simulink model "bolita_sim_2018a"  (R2018a)
settings: Solver=VariableStepAuto  StartTime=0.0  StopTime=10  RelTol=1e-3
values from neighbouring files (symbols this model uses):
  A = double(subs(A,{x1,x2,x3,u},{x1_eq,x2_eq,x3_eq,u_eq}))    [bolita.m]
  B = double(subs(B,{x1,x2,x3,u},{x1_eq,x2_eq,x3_eq,u_eq}))    [bolita.m]
  C = double(subs(C,{x1,x2,x3,u},{x1_eq,x2_eq,x3_eq,u_eq}))    [bolita.m]
  Ki = Ki(end)    [bolita.m]
  Ksr = Ki(1:3)    [bolita.m]
  L = (acker(A',C',[-200 -200 -200]))'    [bolita.m]
  u_eq = double(solve(subs(x3_dot,x3,x3_eq)))    [bolita.m]
  x1_eq = 0    [bolita.m]
  x2_eq = 0    [bolita.m]
  x3_eq = double(solve(subs(x2_dot,x1,x1_eq)))    [bolita.m]
settings Model: Creator=Carlos  LastModifiedBy=Carlos
settings DebuggingCC: LibraryContextMissingDiagnostic=warning
settings SFSimCC: SimUseLocalCustomCode=on
settings RTWCC: RTWUseLocalCustomCode=on

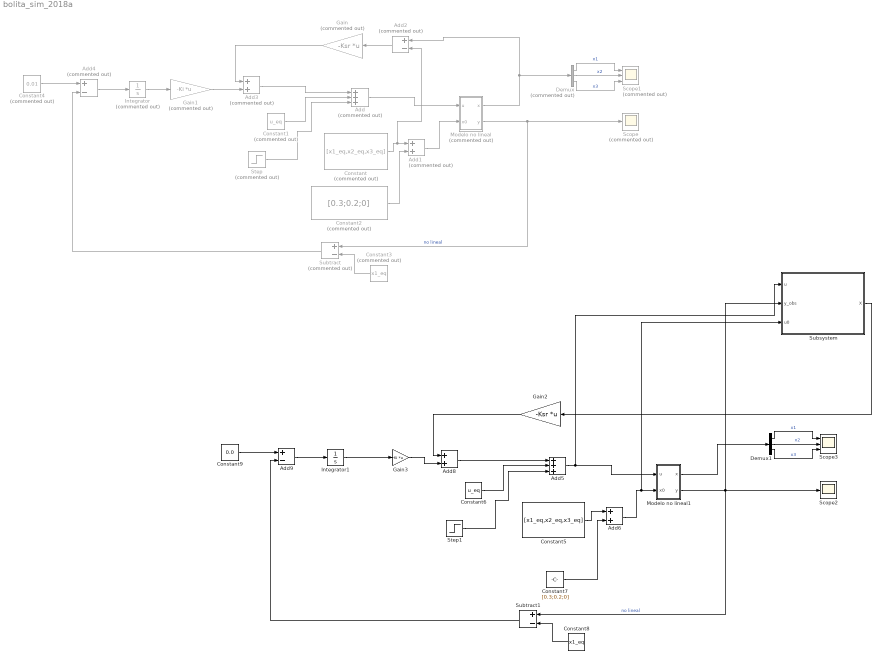
== system bolita_sim_2018a ==
  Add : Sum  Commented=on  Inputs=+++
  Add1 : Sum  Commented=on
  Add2 : Sum  Commented=on  Inputs=+-
  Add3 : Sum  Commented=on
  Add4 : Sum  Commented=on  Inputs=+-
  Add5 : Sum  Inputs=+++
  Add6 : Sum
  Add8 : Sum
  Add9 : Sum  Inputs=+-
  Constant : Constant  Commented=on  Value=[x1_eq,x2_eq,x3_eq]
  Constant1 : Constant  Commented=on  Value=u_eq
  Constant2 : Constant  Commented=on  Value=[0.3;0.2;0]
  Constant3 : Constant  Commented=on  Value=x1_eq
  Constant4 : Constant  Commented=on  Value=0.01
  Constant5 : Constant  Value=[x1_eq,x2_eq,x3_eq]
  Constant6 : Constant  Value=u_eq
  Constant7 : Constant  Value=[0.3;0.2;0]
  Constant8 : Constant  Value=x1_eq
  Constant9 : Constant  Value=0.0
  Demux : Demux  Commented=on  Outputs=3
  Demux1 : Demux  Outputs=3
  Gain : Gain  Commented=on  Gain=-Ksr  Multiplication=Matrix(K*u) (u vector)
  Gain1 : Gain  Commented=on  Gain=-Ki  Multiplication=Matrix(K*u) (u vector)
  Gain2 : Gain  Gain=-Ksr  Multiplication=Matrix(K*u) (u vector)
  Gain3 : Gain  Gain=-Ki  Multiplication=Matrix(K*u) (u vector)
  Integrator : Integrator  Commented=on
  Integrator1 : Integrator
  Modelo no lineal : Subsystem  Commented=on
  Modelo no lineal1 : Subsystem
  Scope : Scope  Commented=on
  Scope1 : Scope  Commented=on  NumInputPorts=3
  Scope2 : Scope
  Scope3 : Scope  NumInputPorts=3
  Step : Step  Commented=on  Time=5  After=300  SampleTime=0
  Step1 : Step  Time=5  After=300  SampleTime=0
  Subsystem : Subsystem
  Subtract : Sum  Commented=on  Inputs=+-
  Subtract1 : Sum  Inputs=+-
  wires:
  Add/1 -> Modelo no lineal/1(u)
  Constant1/1 -> Add/2
  Modelo no lineal/1(x) -> Demux/1, Add2/1
  Constant/1 -> Add2/2, Add1/1
  Add1/1 -> Modelo no lineal/2(x0)
  Constant2/1 -> Add1/2
  Add2/1 -> Gain/1
  Modelo no lineal/2(y) -> Subtract/1, Scope/1  "no lineal"
  Demux/1 -> Scope1/1  "x1"
  Demux/2 -> Scope1/2  "x2"
  Demux/3 -> Scope1/3  "x3"
  Add3/1 -> Add/1
  Gain1/1 -> Add3/2
  Gain/1 -> Add3/1
  Integrator/1 -> Gain1/1
  Constant3/1 -> Subtract/2
  Add4/1 -> Integrator/1
  Subtract/1 -> Add4/2
  Constant4/1 -> Add4/1
  Step/1 -> Add/3
  Subsystem/1(X) -> Gain2/1
  Add8/1 -> Add5/1
  Step1/1 -> Add5/3
  Add9/1 -> Integrator1/1
  Demux1/3 -> Scope3/3  "x3"
  Integrator1/1 -> Gain3/1
  Constant8/1 -> Subtract1/2
  Constant9/1 -> Add9/1
  Gain2/1 -> Add8/1
  Gain3/1 -> Add8/2
  Modelo no lineal1/1(x) -> Demux1/1
  Subtract1/1 -> Add9/2
  Modelo no lineal1/2(y) -> Subsystem/2("y_obs "), Subtract1/1, Scope2/1  "no lineal"
  Demux1/1 -> Scope3/1  "x1"
  Demux1/2 -> Scope3/2  "x2"
  Constant5/1 -> Add6/1
  Add6/1 -> Subsystem/3(u0), Modelo no lineal1/2(x0)
  Constant7/1 -> Add6/2
  Add5/1 -> Subsystem/1(u), Modelo no lineal1/1(u)
  Constant6/1 -> Add5/2

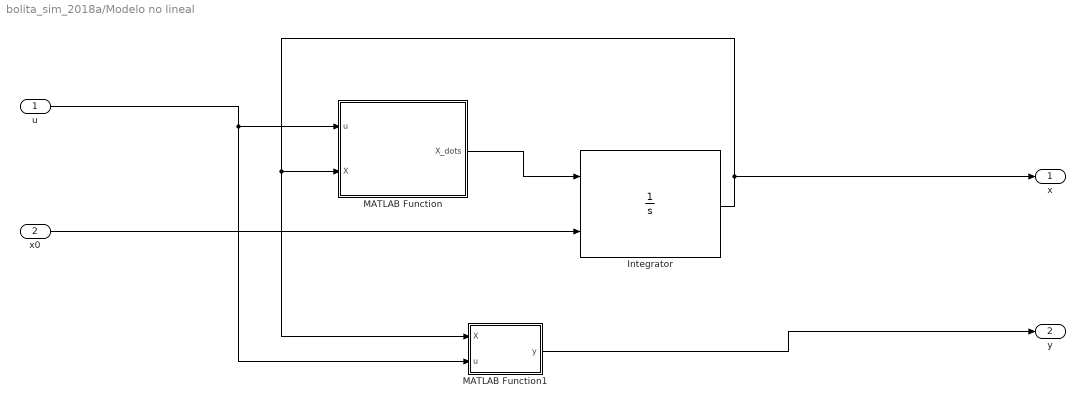
== system bolita_sim_2018a/Modelo no lineal ==
  u : Inport
  x0 : Inport  Port=2
  Integrator : Integrator  InitialConditionSource=external
  MATLAB Function : MATLAB Function  TreatAsAtomicUnit=on
  MATLAB Function1 : MATLAB Function  TreatAsAtomicUnit=on
  x : Outport
  y : Outport  Port=2
  wires:
  Integrator/1 -> x/1, MATLAB Function1/1(X), MATLAB Function/2(X)
  u/1 -> MATLAB Function1/2(u), MATLAB Function/1(u)
  MATLAB Function/1(X_dots) -> Integrator/1
  MATLAB Function1/1(y) -> y/1
  x0/1 -> Integrator/2

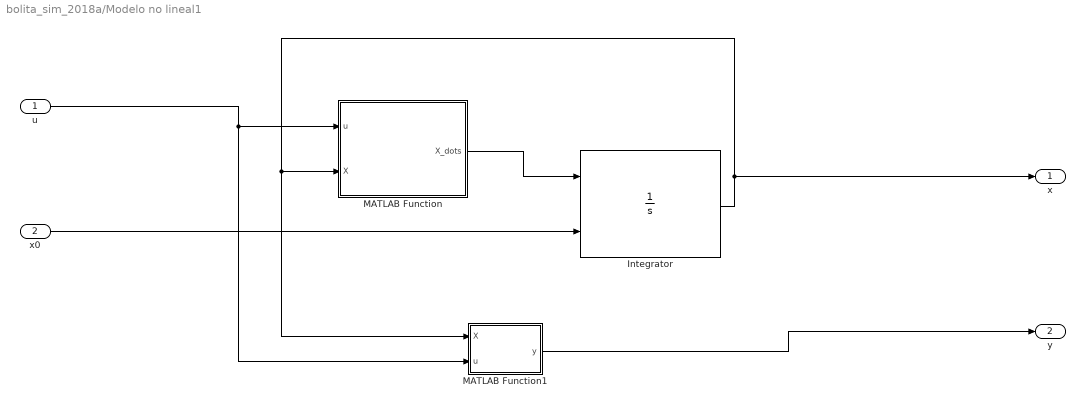
== system bolita_sim_2018a/Modelo no lineal1 ==
  u : Inport
  x0 : Inport  Port=2
  Integrator : Integrator  InitialConditionSource=external
  MATLAB Function : MATLAB Function  TreatAsAtomicUnit=on
  MATLAB Function1 : MATLAB Function  TreatAsAtomicUnit=on
  x : Outport
  y : Outport  Port=2
  wires:
  Integrator/1 -> x/1, MATLAB Function1/1(X), MATLAB Function/2(X)
  u/1 -> MATLAB Function1/2(u), MATLAB Function/1(u)
  MATLAB Function/1(X_dots) -> Integrator/1
  MATLAB Function1/1(y) -> y/1
  x0/1 -> Integrator/2

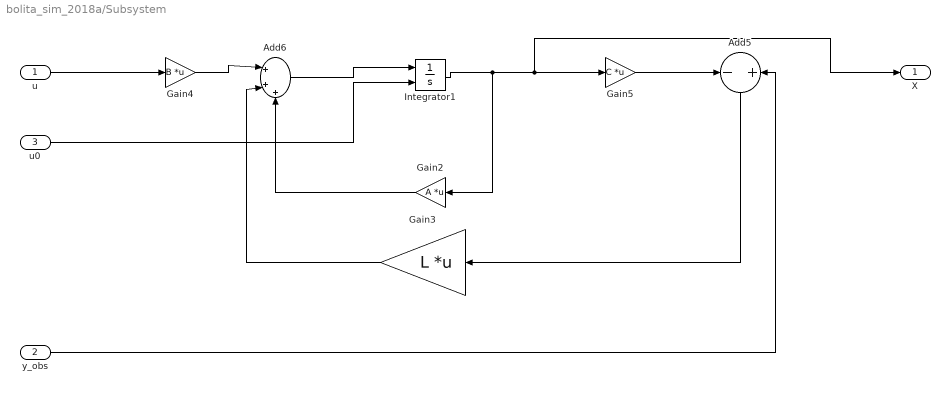
== system bolita_sim_2018a/Subsystem ==
  u : Inport
  "y_obs " : Inport  Port=2
  u0 : Inport  Port=3
  Add5 : Sum  Inputs=-|+
  Add6 : Sum  Inputs=|+++
  Gain2 : Gain  Gain=A  Multiplication=Matrix(K*u) (u vector)
  Gain3 : Gain  Gain=L  Multiplication=Matrix(K*u) (u vector)
  Gain4 : Gain  Gain=B  Multiplication=Matrix(K*u) (u vector)
  Gain5 : Gain  Gain=C  Multiplication=Matrix(K*u) (u vector)
  Integrator1 : Integrator  InitialConditionSource=external
  X : Outport
  wires:
  u/1 -> Gain4/1
  Gain5/1 -> Add5/1
  Gain3/1 -> Add6/2
  "y_obs "/1 -> Add5/2
  Integrator1/1 -> Gain2/1, X/1, Gain5/1
  Add5/1 -> Gain3/1
  Add6/1 -> Integrator1/1
  Gain2/1 -> Add6/3
  Gain4/1 -> Add6/1
  u0/1 -> Integrator1/2

== matlab function bolita_sim_2018a/Modelo no lineal/MATLAB Function1 ==
  data: X input; u input; y output
function  y = fcn(X,u)

y = X(1);

== matlab function bolita_sim_2018a/Modelo no lineal/MATLAB Function ==
  data: u input; X_dots output; X input
function X_dots = fcn(u,X)

R=4;
L=1;
m=0.2;
g=10;

x1 = X(1);
x2= X(2);
x3 = X(3);
F1=0.5*(((2+x3)^2)/((1-x1)^2));
F2=0.5*(((2-x3)^2)/((1+x1)^2));
x2_dot = -g+(F1-F2)/m;
x1_dot = x2;
x3_dot = -(x3*abs(x3))/(L/R)+u/L;


X_dots =[x1_dot x2_dot x3_dot];

== matlab function bolita_sim_2018a/Modelo no lineal1/MATLAB Function ==
  data: u input; X_dots output; X input
function X_dots = fcn(u,X)

R=4;
L=1;
m=0.2;
g=10;

x1 = X(1);
x2= X(2);
x3 = X(3);
F1=0.5*(((2+x3)^2)/((1-x1)^2));
F2=0.5*(((2-x3)^2)/((1+x1)^2));
x2_dot = -g+(F1-F2)/m;
x1_dot = x2;
x3_dot = -(x3*abs(x3))/(L/R)+u/L;


X_dots =[x1_dot x2_dot x3_dot];

== matlab function bolita_sim_2018a/Modelo no lineal1/MATLAB Function1 ==
  data: X input; u input; y output
function  y = fcn(X,u)

y = X(1);
